simulink model "aerosonde_demo4"  (Simulink 4.0)
settings: Solver=ode4  StartTime=0.0  StopTime=90  FixedStep=0.02  RelTol=1e-3
libraries: simulink_extras x3, aerosimlib x1
settings Model: LastModifiedBy=mariusn  SaveTime=off  SaveOutput=off  LimitDataPoints=off  UnconnectedInputMsg=none  UnconnectedOutputMsg=none  UnconnectedLineMsg=none  BlockReductionOpt=off

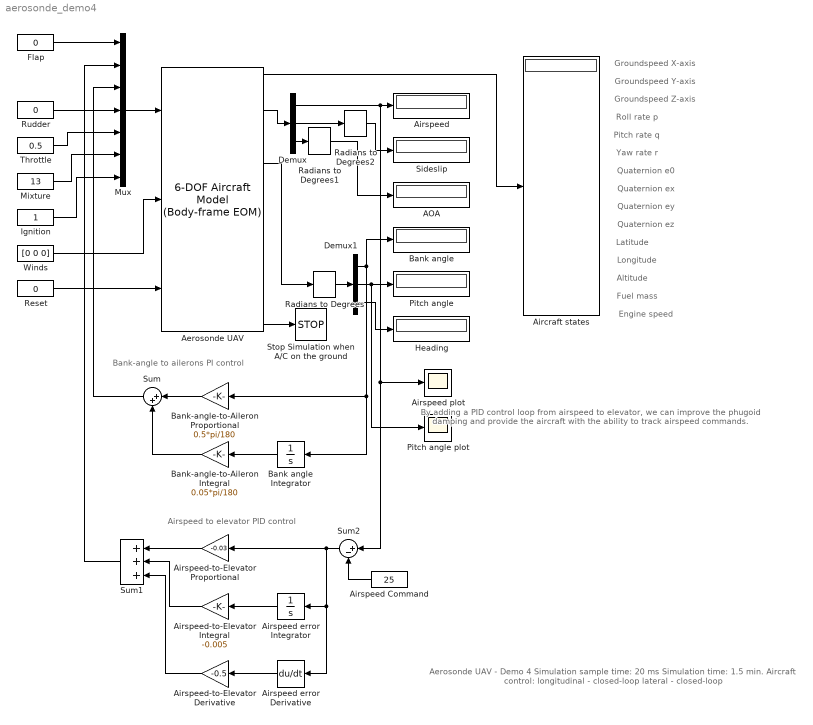
== system aerosonde_demo4 ==
  note: Groundspeed X-axis
  note: Groundspeed Y-axis
  note: Groundspeed Z-axis
  note: Roll rate p
  note: Pitch rate q
  note: Yaw rate r
  note: Quaternion e0
  note: Quaternion ex
  note: Quaternion ey
  note: Quaternion ez
  note: Latitude
  note: Longitude
  note: Altitude
  note: Fuel mass
  note: Engine speed
  note: Aerosonde UAV - Demo 4
      | Simulation sample time: 20 ms
      | Simulation time: 1.5 min.
      | Aircraft control: longitudinal - closed-loop
      |                  lateral - closed-loop
  note: Bank-angle to ailerons PI control
  note: By adding a PID control loop from airspeed to elevator,
      | we can improve the phugoid damping and provide the
      | aircraft with the ability to track airspeed commands.
  note: Airspeed to elevator PID control
  AOA : Display
      settings: Format=short
  Aerosonde UAV : aerosimlib/Complete Aircraft/6-DOF Aircraft Model (Body-frame EOM)  aircraftcfg='aerosondecfg.mat'  VelocitiesIni=[23 0 0]'  RatesIni=[0 0 0]'  QuaternionsIni=[1 0 0 0]'  PositionIni=[45*pi/180 -122*pi/180 1000]'  FuelIni=2  OmegaIni=5000*pi/30  GndAlt=20  wmmfile='C:\Program Files\AeroSim\wmm.cof'  dmy=[09 01 2002]  tsamp=0.02
  Aircraft states : Display
      settings: Format=short
  Airspeed : Display
      settings: Format=short
  Airspeed Command : Constant  Orientation=left  Value=25
  Airspeed error Derivative : Derivative  Orientation=left
  Airspeed error Integrator : Integrator  Orientation=left  ExternalReset=none  InitialConditionSource=internal  InitialCondition=0  LimitOutput=off  UpperSaturationLimit=inf  LowerSaturationLimit=-inf  ShowSaturationPort=off  ShowStatePort=off  AbsoluteTolerance=auto
  Airspeed plot : Scope
      settings: TimeRange=90  YMin=23  YMax=26.5  SaveToWorkspace=off  SaveName=ScopeData  MaxDataPoints=5000
  Airspeed-to-Elevator Derivative : Gain  Orientation=left  Gain=-0.5  Multiplication=Element-wise(K.*u)  SaturateOnIntegerOverflow=on
  Airspeed-to-Elevator Integral : Gain  Orientation=left  Gain=-0.005  Multiplication=Element-wise(K.*u)  SaturateOnIntegerOverflow=on
  Airspeed-to-Elevator Proportional : Gain  Orientation=left  Gain=-0.03  Multiplication=Element-wise(K.*u)  SaturateOnIntegerOverflow=on
  Bank angle : Display
      settings: Format=short
  Bank angle Integrator : Integrator  Orientation=left  ExternalReset=none  InitialConditionSource=internal  InitialCondition=0  LimitOutput=off  UpperSaturationLimit=inf  LowerSaturationLimit=-inf  ShowSaturationPort=off  ShowStatePort=off  AbsoluteTolerance=auto
  Bank-angle-to-Aileron Integral : Gain  Orientation=left  Gain=0.05*pi/180  Multiplication=Element-wise(K.*u)  SaturateOnIntegerOverflow=on
  Bank-angle-to-Aileron Proportional : Gain  Orientation=left  Gain=0.5*pi/180  Multiplication=Element-wise(K.*u)  SaturateOnIntegerOverflow=on
  Demux : Demux  Outputs=3  BusSelectionMode=off
  Demux1 : Demux  Outputs=3  BusSelectionMode=off
  Flap : Constant  Value=0
  Heading : Display
      settings: Format=short
  Ignition : Constant  Value=1
  Mixture : Constant  Value=13
  Mux : Mux  Inputs=7
  Pitch angle : Display
      settings: Format=short
  Pitch angle plot : Scope
      settings: TimeRange=90  YMin=0  YMax=3.5  SaveToWorkspace=off  MaxDataPoints=5000
  Radians to Degrees : simulink_extras/Transformations/Radians to Degrees
  Radians to Degrees1 : simulink_extras/Transformations/Radians to Degrees
  Radians to Degrees2 : simulink_extras/Transformations/Radians to Degrees
  Reset : Constant  Value=0
  Rudder : Constant  Value=0
  Sideslip : Display
      settings: Format=short
  Stop Simulation when A/C on the ground : Stop
  Sum : Sum  Orientation=left  Inputs=|++  SaturateOnIntegerOverflow=on
  Sum1 : Sum  Orientation=left  Inputs=+++  SaturateOnIntegerOverflow=on
  Sum2 : Sum  Orientation=left  Inputs=|+-  SaturateOnIntegerOverflow=on
  Throttle : Constant  Value=0.5
  Winds : Constant  Value=[0 0 0]
  wires:
  Reset/1 -> Aerosonde UAV/3
  Winds/1 -> Aerosonde UAV/2
  Aerosonde UAV/1 -> Aircraft states/1
  Aerosonde UAV/6 -> Radians to Degrees/1
  Aerosonde UAV/3 -> Demux/1
  Demux/3 -> Radians to Degrees1/1
  Demux/2 -> Radians to Degrees2/1
  Demux/1 -> Airspeed/1, Airspeed plot/1, Sum2/1
  Radians to Degrees2/1 -> Sideslip/1
  Radians to Degrees1/1 -> AOA/1
  Aerosonde UAV/15 -> Stop Simulation when A/C on the ground/1
  Radians to Degrees/1 -> Demux1/1
  Demux1/2 -> Pitch angle/1, Pitch angle plot/1
  Demux1/3 -> Heading/1
  Demux1/1 -> Bank angle/1, Bank-angle-to-Aileron Proportional/1, Bank angle Integrator/1
  Flap/1 -> Mux/1
  Rudder/1 -> Mux/4
  Throttle/1 -> Mux/5
  Mixture/1 -> Mux/6
  Ignition/1 -> Mux/7
  Mux/1 -> Aerosonde UAV/1
  Bank-angle-to-Aileron Proportional/1 -> Sum/1
  Bank angle Integrator/1 -> Bank-angle-to-Aileron Integral/1
  Bank-angle-to-Aileron Integral/1 -> Sum/2
  Sum/1 -> Mux/3
  Airspeed error Derivative/1 -> Airspeed-to-Elevator Derivative/1
  Airspeed error Integrator/1 -> Airspeed-to-Elevator Integral/1
  Airspeed-to-Elevator Proportional/1 -> Sum1/1
  Airspeed-to-Elevator Integral/1 -> Sum1/2
  Airspeed-to-Elevator Derivative/1 -> Sum1/3
  Sum1/1 -> Mux/2
  Sum2/1 -> Airspeed-to-Elevator Proportional/1, Airspeed error Integrator/1, Airspeed error Derivative/1
  Airspeed Command/1 -> Sum2/2
